simulink model "PubIfDecisionLM_MDL"  (R2020b)
settings: configuration reference "DspaceConfig" (kept outside this file)
PostLoadFcn:
  | if any(exist('dsrtsu_mdlpostloadfcn', 'file') ~= 0), dsrtsu_mdlpostloadfcn('Execute', bdroot); end
InitFcn:
  | , if any(exist('dsmpb_private', 'file') ~= 0), dsmpb_private('dsmpb_mdlclblib', 'Init', bdroot); end,
undefined symbols (not defined in the file or in its folder): OFM_OBJ_FUSIONTYPE_E, OFM_OBJ_MOVINGSTATE_E, OFM_OBJ_ORIENTATION_E, OFM_OBJ_TYPE_E, P_LM_Cyc, P_LM_EMLHistKapRcdBufSize, P_LM_EMLHistTrajBaseDis, P_LM_EMLHistTrajPNum, P_LM_EMLKapCorrMaxThre, P_LM_EMLMinKapThre, P_LM_EMLPathDisDiffThre, P_LM_EMLQuaFiltPar, P_LM_EMLTurnActKapThre, P_LM_EMLValidQuaThre, P_LM_FntPath1Disgap, P_LM_FntPath1MinDis, P_LM_FntPath1Timegap, P_LM_FntPath2Disgap, P_LM_FntPath2MinDis, P_LM_FntPath2Timegap, P_LM_FntPath3Disgap, P_LM_FntPath3MinDis, P_LM_FntPath3Timegap, P_LM_FusBLParFiltP, P_LM_FusEVDifC2Thre, P_LM_FusEVOPath1AllVSLDisThre, P_LM_FusEVOPath1AllVSLLostNumThre, P_LM_FusEVOPath1AllVSLQuaThre, P_LM_FusEVOPath1OTLFacNLC, P_LM_FusOTLQuaThre, P_LM_FusOTLSW, P_LM_FusParC0Index, P_LM_FusParC1Index, P_LM_FusParC2Index, P_LM_FusParC3Index, P_LM_FusVSLQuaThre, P_LM_FusVSLSW, P_LM_FusVSLValidSteerWheerAngThre, P_LM_FusVSLValidVxvThre, P_LM_LaneWidth, P_LM_OTLBufTPInfoEvaFactor, P_LM_OTLObjNum, P_LM_OTLObjSelectAgeThre, P_LM_OTLObjSelectDxAssessVx, P_LM_OTLObjSelectDxThre, P_LM_OTLObjSelectVxThre, P_LM_OTLObjSelectVyAssessDx, P_LM_OTLObjSelectVyThre, P_LM_OTLTrajPntBaseDis, P_LM_OTLTrajStdThre, P_LM_VSLAvailLineNum, P_LM_VSLBLSDiffThre, P_LM_VSLBLSDisRatio, P_LM_VSLFusBLParFiltP_C1, P_LM_VSLFusBLParFiltP_C2, P_LM_VSLFusBLParFiltP_C3, P_LM_VSLFusBLParFiltP_Quality, P_LM_VSLHistTrajBaseDis, P_LM_VSLHistTrajPNum, P_LM_VSLLCC0diff ... (+18)
libraries: simulink x145, LM_LIB x43
(part 14 of 24)

== system PubIfDecisionLM_MDL/Subsystem2/LM_VSL/LM_VSLFntPath/LM_VSL_LineInfoEvalutaion/LM_VSL_BaseLinePCalc3/Subsystem1 ==
  LM_VSLBaseC1 : Inport
  LM_VSLBaseC2 : Inport  Port=2
  LM_VSLBaseC3 : Inport  Port=3
  LM_VSLBaseQuality : Inport  Port=4
  Add{1..3,12} (4 alike) : Sum
  Constant1 : Constant  Value=P_LM_VSLFusBLParFiltP_C2  OutDataTypeStr=single
  Constant10 : Constant  Value=P_LM_VSLFusBLParFiltP_C1  OutDataTypeStr=single
  Constant2 : Constant  Value=P_LM_VSLFusBLParFiltP_C3  OutDataTypeStr=single
  Constant3 : Constant  Value=P_LM_VSLFusBLParFiltP_Quality  OutDataTypeStr=single
  Data Type Conversion : DataTypeConversion  OutDataTypeStr=single
  Product{1..3,17} (4 alike) : Product
  Subtract{1..4} (4 alike) : Sum  Inputs=+-
  Unit Delay{1..4} (4 alike) : UnitDelay  SampleTime=-1  HasFrameUpgradeWarning=on
  LM_VSLBaseC1Filt : Outport
  LM_VSLBaseC2Filt : Outport  Port=2
  LM_VSLBaseC3Filt : Outport  Port=3
  LM_VSLBaseQualityFilt : Outport  Port=4
  wires:
  Data Type Conversion/1 -> LM_VSLBaseQualityFilt/1
  LM_VSLBaseQuality/1 -> Subtract4/1
  Product3/1 -> Add3/1
  Subtract4/1 -> Product3/1
  Unit Delay4/1 -> Subtract4/2, Add3/2
  Constant3/1 -> Product3/2
  Add3/1 -> Unit Delay4/1, Data Type Conversion/1
  Add2/1 -> Unit Delay3/1, LM_VSLBaseC3Filt/1
  Constant2/1 -> Product2/2
  Unit Delay3/1 -> Add2/2, Subtract3/2
  Subtract3/1 -> Product2/1
  Product2/1 -> Add2/1
  LM_VSLBaseC3/1 -> Subtract3/1
  LM_VSLBaseC2/1 -> Subtract1/1
  Product1/1 -> Add1/1
  Subtract1/1 -> Product1/1
  Unit Delay1/1 -> Subtract1/2, Add1/2
  Constant1/1 -> Product1/2
  Constant10/1 -> Product17/2
  Unit Delay2/1 -> Add12/2, Subtract2/2
  Subtract2/1 -> Product17/1
  Product17/1 -> Add12/1
  LM_VSLBaseC1/1 -> Subtract2/1
  Add12/1 -> LM_VSLBaseC1Filt/1, Unit Delay2/1
  Add1/1 -> Unit Delay1/1, LM_VSLBaseC2Filt/1

== system PubIfDecisionLM_MDL/Subsystem2/LM_VSL/LM_VSLFntPath/LM_VSL_LineInfoEvalutaion/LM_VSL_LineInfoEvalutaion/LM_VSL_LineDiffEvalutaion ==
  LM_VSLLineExistVect : Inport
  LM_VSLLineQualityVect : Inport  Port=2
  LM_VSLLineDisFntVect : Inport  Port=3
  LM_ComLineLostNum : Inport  Port=4
  LM_VSLLineC0Vect : Inport  Port=5
  LM_VSLLineC1Vect : Inport  Port=6
  LM_VSLLineC2Vect : Inport  Port=7
  LM_VSLLineC3Vect : Inport  Port=8
  LM_VSLLineMaxQuality : Inport  Port=9
  LM_VSLLineMaxDis : Inport  Port=10
  LM_VSLLineMaxDisIndex : Inport  Port=11
  LM_VSLLineMaxQualityIndex : Inport  Port=12
  Constant : Constant  Value=P_LM_VSLBLSDiffThre  OutDataTypeStr=single
  Constant1 : Constant  Value=P_LM_VSLBLSDisRatio  OutDataTypeStr=single
  LM_VSL_BaseLineSelc : MATLAB Function  TreatAsAtomicUnit=on
  LM_VSL_DiffMaxLineEvaluation3 : MATLAB Function  TreatAsAtomicUnit=on
  Terminator : Terminator
  "Diffnum " : Outport
  LM_VSLDiffValid : Outport  Port=2
  LM_VSLBLFntDis : Outport  Port=3
  wires:
  Constant1/1 -> LM_VSL_DiffMaxLineEvaluation3/11(P_LM_VSLBLSDisRatio)
  Constant/1 -> LM_VSL_DiffMaxLineEvaluation3/10(P_LM_VSLBLSDiffThre)
  LM_VSL_DiffMaxLineEvaluation3/2(LM_VSLDiffValue) -> Terminator/1  "LM_VSLDiffValue"
  LM_VSL_BaseLineSelc/2(LM_VSLBLFntDis) -> LM_VSL_DiffMaxLineEvaluation3/2(LM_VSLBLFntDis), LM_VSLBLFntDis/1
  LM_VSL_DiffMaxLineEvaluation3/3(Diffnum) -> "Diffnum "/1
  [LM_VSLLineDisFntVect] -> LM_VSL_DiffMaxLineEvaluation3/9(LM_VSLLineDisFntVect)
  LM_VSL_DiffMaxLineEvaluation3/1(LM_VSLDiffValid) -> LM_VSLDiffValid/1
  LM_VSLLineC2Vect/1 -> LM_VSL_DiffMaxLineEvaluation3/7(LM_VSLLineC2Vect)
  LM_VSLLineQualityVect/1 -> LM_VSL_BaseLineSelc/1(LM_VSLLineQualityVect)
  LM_ComLineLostNum/1 -> LM_VSL_DiffMaxLineEvaluation3/5(LM_ComLineLostNum)
  LM_VSLLineExistVect/1 -> LM_VSL_BaseLineSelc/7(LM_VSLLineExistVect), LM_VSL_DiffMaxLineEvaluation3/3(LM_VSLLineExistVect)
  LM_VSL_BaseLineSelc/1(LM_VSLBLIndex) -> LM_VSL_DiffMaxLineEvaluation3/1(LM_VSLBLIndex)  "LM_VSLBLIndex"
  LM_VSLLineC0Vect/1 -> LM_VSL_DiffMaxLineEvaluation3/4(LM_VSLLineC0Vect)
  LM_VSLLineC1Vect/1 -> LM_VSL_DiffMaxLineEvaluation3/6(LM_VSLLineC1Vect)
  LM_VSLLineC3Vect/1 -> LM_VSL_DiffMaxLineEvaluation3/8(LM_VSLLineC3Vect)
  LM_VSLLineDisFntVect/1 -> LM_VSL_BaseLineSelc/2(LM_VSLLineDisFntVect), [LM_VSLLineDisFntVect]
  LM_VSLLineMaxDis/1 -> LM_VSL_BaseLineSelc/3(LM_VSLLineMaxDis)
  LM_VSLLineMaxDisIndex/1 -> LM_VSL_BaseLineSelc/4(LM_VSLLineMaxDisIndex)
  LM_VSLLineMaxQuality/1 -> LM_VSL_BaseLineSelc/5(LM_VSLLineMaxQuality)
  LM_VSLLineMaxQualityIndex/1 -> LM_VSL_BaseLineSelc/6(LM_VSLLineMaxQualityIndex)

== system PubIfDecisionLM_MDL/Subsystem2/LM_VSL/LM_VSLFntPath/LM_VSL_LineInfoEvalutaion/LM_VSL_LineInfoEvalutaion/LM_VSL_LineDisEvaluation ==
  LM_ComAllLineLost_flg : Inport
  LM_VSLLineExistVect : Inport  Port=2
  LM_VSLLineDisFntVect : Inport  Port=3
  If : If  IfExpression=u1 == 1
  If Action Subsystem : Subsystem  TreatAsAtomicUnit=on
  If Action Subsystem1 : Subsystem  TreatAsAtomicUnit=on
  Merge{,1..3} (4 alike) : Merge
  Terminator1 : Terminator
  Terminator2 : Terminator
  LM_VSLLineMaxDis : Outport
  LM_VSLLineMaxDisIndex : Outport  Port=2
  wires:
  Merge3/1 -> Terminator2/1
  If Action Subsystem1/4(LM_VSLLineMeanDis) -> Merge3/2
  If Action Subsystem/4(LM_VSLLineMeanDis) -> Merge3/1
  LM_ComAllLineLost_flg/1 -> If/1
  If/1 -> If Action Subsystem/Action
  If/2 -> If Action Subsystem1/Action
  LM_VSLLineExistVect/1 -> If Action Subsystem1/1(LM_VSLLineExistVect)
  LM_VSLLineDisFntVect/1 -> If Action Subsystem1/2(LM_VSLLineDisFntVect)
  If Action Subsystem/1(LM_VSLLineMaxDis) -> Merge/1
  If Action Subsystem1/1(LM_VSLLineMaxDis) -> Merge/2
  Merge/1 -> LM_VSLLineMaxDis/1
  If Action Subsystem1/2(LM_VSLLineMaxDisIndex) -> Merge1/2
  If Action Subsystem/2(LM_VSLLineMaxDisIndex) -> Merge1/1
  Merge1/1 -> LM_VSLLineMaxDisIndex/1
  If Action Subsystem/3(LM_VSLLineDisSortIndexVect) -> Merge2/1
  Merge2/1 -> Terminator1/1
  If Action Subsystem1/3(LM_VSLLineDisSortIndexVect) -> Merge2/2

== system PubIfDecisionLM_MDL/Subsystem2/LM_VSL/LM_VSLFntPath/LM_VSL_LineInfoEvalutaion/LM_VSL_LineInfoEvalutaion/LM_VSL_LineQualityEvalutaion ==
  LM_ComAllLineLost_flg : Inport
  LM_VSLLineExistVect : Inport  Port=2
  LM_VSLLineQualityVect : Inport  Port=3
  If : If  IfExpression=u1 == 1
  If Action Subsystem : Subsystem  TreatAsAtomicUnit=on
  If Action Subsystem1 : Subsystem  TreatAsAtomicUnit=on
  LM_VSLMinQualityLineValidJudge : Subsystem
  Merge{,1..5} (6 alike) : Merge
  Terminator2 : Terminator
  LM_VSLLineMinQualityIndex : Outport
  LM_VSLLineMaxQualityIndex : Outport  Port=2
  LM_VSLLineMaxQuality : Outport  Port=3
  LM_VSLMinQualityLineValid : Outport  Port=4
  wires:
  If/1 -> If Action Subsystem/Action
  If/2 -> If Action Subsystem1/Action
  LM_ComAllLineLost_flg/1 -> If/1
  LM_VSLLineQualityVect/1 -> If Action Subsystem1/2(LM_VSLLineQualityVect)
  LM_VSLLineExistVect/1 -> If Action Subsystem1/1(LM_VSLLineExistVect)
  If Action Subsystem/1(LM_VSLLineMaxQuality) -> Merge/1
  If Action Subsystem/2(LM_VSLLineMaxQualityIndex) -> Merge1/1
  If Action Subsystem/4(LM_VSLLineMinQuality) -> Merge2/1
  If Action Subsystem/3(LM_VSLLineMinQualityIndex) -> Merge3/1
  If Action Subsystem/5(LM_VSLLineMeanQuality) -> Merge4/1
  If Action Subsystem/6(LM_VSLLineQualityVar) -> Merge5/1
  Merge/1 -> LM_VSLLineMaxQuality/1  "LM_VSLLineMaxQuality"
  Merge1/1 -> LM_VSLLineMaxQualityIndex/1  "LM_VSLLineMaxQualityIndex"
  Merge2/1 -> LM_VSLMinQualityLineValidJudge/1(LM_VSLLineMinQuality)  "LM_VSLLineMinQuality"
  Merge3/1 -> LM_VSLLineMinQualityIndex/1  "LM_VSLLineMinQualityIndex"
  Merge4/1 -> LM_VSLMinQualityLineValidJudge/2(LM_VSLLineMeanQuality)  "LM_VSLLineMeanQuality"
  Merge5/1 -> Terminator2/1
  If Action Subsystem1/1(LM_VSLLineMaxQuality) -> Merge/2
  If Action Subsystem1/2(LM_VSLLineMaxQualityIndex) -> Merge1/2
  If Action Subsystem1/4(LM_VSLLineMinQuality) -> Merge2/2
  If Action Subsystem1/3(LM_VSLLineMinQualityIndex) -> Merge3/2
  If Action Subsystem1/5(LM_VSLLineMeanQuality) -> Merge4/2
  If Action Subsystem1/6(LM_VSLLineQualityVar) -> Merge5/2
  LM_VSLMinQualityLineValidJudge/1(LM_VSLMinQualityLineValid) -> LM_VSLMinQualityLineValid/1

== system PubIfDecisionLM_MDL/Subsystem2/LM_VSL/LM_VSLRearPath/LM_VSLHistLineInfoCoordinateConvert/If Action Subsystem/For Each Subsystem ==
  LM_EMLOffsetX : Inport
  LM_EMLOffsetY : Inport  Port=2
  LM_EMLOffsetAng : Inport  Port=3
  LM_VSLLRC0HistInfoXK1 : Inport  Port=4  Partition=on  PartitionDimension=1  PartitionWidth=1  PartitionOffset=0
  LM_VSLLRC0HistInfoYK1 : Inport  Port=5  Partition=on  PartitionDimension=1  PartitionWidth=1  PartitionOffset=0
  LM_VSLRLC0HistInfoXK1 : Inport  Port=6  Partition=on  PartitionDimension=1  PartitionWidth=1  PartitionOffset=0
  LM_VSLRLC0HistInfoYK1 : Inport  Port=7  Partition=on  PartitionDimension=1  PartitionWidth=1  PartitionOffset=0
  For Each : ForEach  DisableCoverage=on
  LM_VSL_LRC0HistInfoConvert : Subsystem
  LM_VSL_RLC0HistInfoConvert : Subsystem
  LM_VSLLRC0HistInfoXK1Adju : Outport  ConcatenationDimension=1
  LM_VSLLRC0HistInfoYK1Adju : Outport  Port=2  ConcatenationDimension=1
  LM_VSLRLC0HistInfoXK1Adju : Outport  Port=3  ConcatenationDimension=1
  LM_VSLRLC0HistInfoYK1Adju : Outport  Port=4  ConcatenationDimension=1
  wires:
  LM_EMLOffsetX/1 -> LM_VSL_RLC0HistInfoConvert/3(LM_EgoVehOffsetX), LM_VSL_LRC0HistInfoConvert/3(LM_EgoVehOffsetX)
  LM_EMLOffsetY/1 -> LM_VSL_RLC0HistInfoConvert/4(LM_EgoVehOffsetY), LM_VSL_LRC0HistInfoConvert/4(LM_EgoVehOffsetY)
  LM_EMLOffsetAng/1 -> LM_VSL_RLC0HistInfoConvert/5(LM_EgoVehOffsetAng), LM_VSL_LRC0HistInfoConvert/5(LM_EgoVehOffsetAng)
  LM_VSL_LRC0HistInfoConvert/1(LM_VSLLLC0HistInfoXK1Adju) -> LM_VSLLRC0HistInfoXK1Adju/1
  LM_VSL_LRC0HistInfoConvert/2(LM_VSLLLC0HistInfoYK1Adju) -> LM_VSLLRC0HistInfoYK1Adju/1
  LM_VSL_RLC0HistInfoConvert/2(LM_VSLLLC0HistInfoYK1Adju) -> LM_VSLRLC0HistInfoYK1Adju/1
  LM_VSL_RLC0HistInfoConvert/1(LM_VSLLLC0HistInfoXK1Adju) -> LM_VSLRLC0HistInfoXK1Adju/1
  LM_VSLLRC0HistInfoYK1/1 -> LM_VSL_LRC0HistInfoConvert/2(LM_VSLLRC0HistInfoYK1)
  LM_VSLLRC0HistInfoXK1/1 -> LM_VSL_LRC0HistInfoConvert/1(LM_VSLLRC0HistInfoXK1)
  LM_VSLRLC0HistInfoYK1/1 -> LM_VSL_RLC0HistInfoConvert/2(LM_VSLRLC0HistInfoYK1)
  LM_VSLRLC0HistInfoXK1/1 -> LM_VSL_RLC0HistInfoConvert/1(LM_VSLRLC0HistInfoXK1)

== system PubIfDecisionLM_MDL/Subsystem2/DIR/DrivingIntentionRecognition1/DIR_LaneChangeProbCalc/DIR_LaneChangeLeftProbCalc/If Action Subsystem/DIR_LaneChgLeProbByC1 ==
  LM_VSLFntPathBaseC1 : Inport
  Constant5 : Constant  Value=-0.035  OutDataTypeStr=single
  Relational Operator5 : RelationalOperator  Operator=<=  OutDataTypeStr=boolean  RndMeth=Nearest
  DIR_LaneChgLeByLineC1Valid : Outport
  wires:
  Constant5/1 -> Relational Operator5/2
  LM_VSLFntPathBaseC1/1 -> Relational Operator5/1
  Relational Operator5/1 -> DIR_LaneChgLeByLineC1Valid/1  "DIR_LaneChgLeByLineC1Valid"

== system PubIfDecisionLM_MDL/Subsystem2/DIR/DrivingIntentionRecognition1/DIR_LaneChangeProbCalc/DIR_LaneChangeLeftProbCalc/If Action Subsystem/DIR_LaneChgLeProbByLaneInfo ==
  LM_LRC0 : Inport
  LM_RLC0 : Inport  Port=2
  DIR_LaneC0DifCalc : Subsystem
  DIR_LaneChgLeProbCalcByLaneBorder : Subsystem
  Unit Delay : UnitDelay  SampleTime=-1  HasFrameUpgradeWarning=on
  DIR_LC2LeProbByLaneBorder : Outport
  wires:
  DIR_LaneC0DifCalc/1(DIR_LaneC0Dif) -> Unit Delay/1, DIR_LaneChgLeProbCalcByLaneBorder/1(DIR_LaneC0Dif)
  Unit Delay/1 -> DIR_LaneC0DifCalc/1(DIR_LaneC0DifK1)
  LM_LRC0/1 -> DIR_LaneChgLeProbCalcByLaneBorder/2(LM_LRC0), DIR_LaneC0DifCalc/2(LM_LRC0)
  LM_RLC0/1 -> DIR_LaneC0DifCalc/3(LM_RLC0)
  DIR_LaneChgLeProbCalcByLaneBorder/1(DIR_LC2LeProbByLaneBorder) -> DIR_LC2LeProbByLaneBorder/1

== system PubIfDecisionLM_MDL/Subsystem2/DIR/DrivingIntentionRecognition1/DIR_LaneChangeProbCalc/DIR_LaneChangeLeftProbCalc/If Action Subsystem/DIR_LaneChgLeProbByLeftTurnSWSts ==
  LeftTurnSWSts : Inport
  Constant : Constant  OutDataTypeStr=uint8
  Constant1 : Constant  OutDataTypeStr=single
  Constant2 : Constant  Value=0  OutDataTypeStr=single
  Relational Operator : RelationalOperator  Operator===  OutDataTypeStr=boolean  RndMeth=Simplest
  Switch : Switch  Criteria=u2 ~= 0
  DIR_LC2LeProbByTurnLampSts : Outport
  wires:
  Switch/1 -> DIR_LC2LeProbByTurnLampSts/1  "DIR_LC2LeProbByTurnLampSts"
  Constant2/1 -> Switch/3
  Constant/1 -> Relational Operator/2
  Relational Operator/1 -> Switch/2
  LeftTurnSWSts/1 -> Relational Operator/1
  Constant1/1 -> Switch/1

== system PubIfDecisionLM_MDL/Subsystem2/DIR/DrivingIntentionRecognition1/DIR_LaneChangeProbCalc/DIR_LaneChangeLeftProbCalc/If Action Subsystem/DIR_LaneChgLeProbCalc ==
  DIR_LC2LeProbBySteer : Inport
  DIR_LC2LeProbByLaneBorder : Inport  Port=2
  DIR_LC2LeProbByTurnLampSts : Inport  Port=3
  DIR_LaneChgLeByLineC1Valid : Inport  Port=4
  Add : Sum
  Add1 : Sum
  Constant : Constant  Value=2  OutDataTypeStr=single
  Constant1 : Constant  Value=0.1  OutDataTypeStr=single
  Constant2 : Constant  Value=0.25  OutDataTypeStr=single
  Constant3 : Constant  Value=0.75  OutDataTypeStr=single
  Constant4 : Constant  Value=0.75  OutDataTypeStr=single
  Divide : Product  Inputs=*/
  Logical Operator : Logic  AllPortsSameDT=off  OutDataTypeStr=boolean
  MinMax : MinMax  Inputs=2
  Product : Product
  Relational Operator : RelationalOperator  Operator=>  OutDataTypeStr=boolean  RndMeth=Simplest
  Relational Operator1 : RelationalOperator  OutDataTypeStr=boolean  RndMeth=Simplest
  Switch : Switch  Criteria=u2 ~= 0
  DIR_tLC2LeValid : Outport
  wires:
  DIR_LC2LeProbBySteer/1 -> Add/1
  DIR_LC2LeProbByLaneBorder/1 -> Add/2
  Add/1 -> Divide/1
  Constant/1 -> Divide/2
  Divide/1 -> MinMax/1
  DIR_LC2LeProbByTurnLampSts/1 -> MinMax/2
  Constant1/1 -> Relational Operator/2
  Relational Operator/1 -> Switch/2
  MinMax/1 -> Switch/3, Product/1, Relational Operator/1
  Constant2/1 -> Product/2
  Product/1 -> Add1/1
  Constant3/1 -> Add1/2
  Add1/1 -> Switch/1
  Switch/1 -> Relational Operator1/1  "DIR_LC2LeProb"
  Constant4/1 -> Relational Operator1/2
  Logical Operator/1 -> DIR_tLC2LeValid/1  "DIR_tLC2LeValid"
  DIR_LaneChgLeByLineC1Valid/1 -> Logical Operator/1
  Relational Operator1/1 -> Logical Operator/2  "DIR_tLC2LeValid"

== system PubIfDecisionLM_MDL/Subsystem2/DIR/DrivingIntentionRecognition1/DIR_LaneChangeProbCalc/DIR_LaneChangeLeftProbCalc/If Action Subsystem/DIR_LaneChgLeProbCalcBySteer ==
  DIR_LeftTurnLampOnTime : Inport
  SteerWheelAngle : Inport  Port=2
  SteerWheelAngleSign : Inport  Port=3
  DIR_LaneChg2LeftProbCalcBySteer : Subsystem
  DIR_LaneChg2LeftProbCalcBySteerWheelAng : Subsystem
  DIR_LaneChg2LeftProbCalcByTurnLampOnTime : Subsystem
  DIR_LC2LeProbBySteer : Outport
  wires:
  DIR_LaneChg2LeftProbCalcBySteerWheelAng/1(DIR_LC2LeProbBySteerWheelAng) -> DIR_LaneChg2LeftProbCalcBySteer/1(DIR_LC2LeProbBySteerWheelAng)
  DIR_LaneChg2LeftProbCalcByTurnLampOnTime/1(DIR_LC2LeProbBytTurnLamp) -> DIR_LaneChg2LeftProbCalcBySteer/2(DIR_LC2LeProbBytTurnLamp)
  DIR_LeftTurnLampOnTime/1 -> DIR_LaneChg2LeftProbCalcByTurnLampOnTime/1(DIR_LeftTurnLampOnTime)
  DIR_LaneChg2LeftProbCalcBySteer/1(DIR_LC2LeProbBySteer) -> DIR_LC2LeProbBySteer/1
  SteerWheelAngle/1 -> DIR_LaneChg2LeftProbCalcBySteerWheelAng/1(SteerWheelAngle)
  SteerWheelAngleSign/1 -> DIR_LaneChg2LeftProbCalcBySteerWheelAng/2(SteerWheelAngleSign)

== system PubIfDecisionLM_MDL/Subsystem2/DIR/DrivingIntentionRecognition1/DIR_LaneChangeProbCalc/DIR_LaneChangeLeftProbCalc/If Action Subsystem1/DIR_LaneChgLeProbByLaneInfo ==
  LM_LRC0 : Inport
  LM_RLC0 : Inport  Port=2
  Abs : Abs
  Abs1 : Abs
  Abs2 : Abs
  Add : Sum
  Constant : Constant  Value=0.8  OutDataTypeStr=single
  Constant1 : Constant  Value=0.05  OutDataTypeStr=single
  Constant2 : Constant  Value=0.1  OutDataTypeStr=single
  Constant3 : Constant  Value=0.6  OutDataTypeStr=single
  Constant4 : Constant  Value=0  OutDataTypeStr=single
  Logical Operator : Logic  Operator=OR  AllPortsSameDT=off  OutDataTypeStr=boolean
  Logical Operator1 : Logic  AllPortsSameDT=off  OutDataTypeStr=boolean
  Logical Operator2 : Logic  Operator=OR  AllPortsSameDT=off  OutDataTypeStr=boolean
  Logical Operator3 : Logic  AllPortsSameDT=off  OutDataTypeStr=boolean
  MinMax : MinMax  Function=max
  Product : Product
  Relational Operator{,1..3} (4 alike) : RelationalOperator  Operator=>  OutDataTypeStr=boolean  RndMeth=Simplest
  Relational Operator4 : RelationalOperator  Operator=<  OutDataTypeStr=boolean  RndMeth=Simplest
  Subtract : Sum  Inputs=+-
  Subtract1 : Sum  Inputs=+-
  Tapped Delay : simulink/Discrete/Tapped Delay  vinit=0.0  samptime=-1  NumDelays=5  DelayOrder=Oldest  includeCurrent=off
  Unit Delay : UnitDelay  SampleTime=-1  HasFrameUpgradeWarning=on
  Unit Delay1 : UnitDelay  SampleTime=-1  HasFrameUpgradeWarning=on
  DIR_LaneChgLeByLaneBorderValid : Outport
  wires:
  Logical Operator3/1 -> DIR_LaneChgLeByLaneBorderValid/1  "DIR_LaneChgLeByLaneBorderValid"
  LM_LRC0/1 -> Add/1, Product/1
  LM_RLC0/1 -> Product/2, Add/2
  Add/1 -> Abs/1
  Unit Delay1/1 -> Subtract1/2
  Unit Delay/1 -> Unit Delay1/1, Subtract/2
  Constant/1 -> Relational Operator/2
  Abs/1 -> Subtract1/1, Subtract/1, Relational Operator/1, Unit Delay/1
  Subtract/1 -> Abs1/1
  Abs1/1 -> Tapped Delay/1, Relational Operator1/1
  Subtract1/1 -> Abs2/1
  Abs2/1 -> Relational Operator2/1
  Constant1/1 -> Relational Operator1/2
  Constant2/1 -> Relational Operator2/2
  Relational Operator1/1 -> Logical Operator/1
  Relational Operator2/1 -> Logical Operator/2
  Tapped Delay/1 -> MinMax/1
  MinMax/1 -> Relational Operator3/1
  Constant3/1 -> Relational Operator3/2
  Product/1 -> Relational Operator4/1
  Constant4/1 -> Relational Operator4/2
  Relational Operator4/1 -> Logical Operator1/1
  Relational Operator/1 -> Logical Operator1/2
  Relational Operator3/1 -> Logical Operator2/1
  Logical Operator/1 -> Logical Operator2/2
  Logical Operator1/1 -> Logical Operator3/1
  Logical Operator2/1 -> Logical Operator3/2

== system PubIfDecisionLM_MDL/Subsystem2/DIR/DrivingIntentionRecognition1/DIR_LaneChangeProbCalc/DIR_LaneChangeLeftProbCalc/If Action Subsystem1/DIR_LaneChgLeProbByLaneInfo1 ==
  LM_VSLFntPathBaseC1 : Inport
  Constant5 : Constant  Value=-0.035  OutDataTypeStr=single
  Relational Operator5 : RelationalOperator  Operator=<=  OutDataTypeStr=boolean  RndMeth=Nearest
  DIR_LaneChgLeByLineC1Valid : Outport
  wires:
  Constant5/1 -> Relational Operator5/2
  LM_VSLFntPathBaseC1/1 -> Relational Operator5/1
  Relational Operator5/1 -> DIR_LaneChgLeByLineC1Valid/1  "DIR_LaneChgLeByLineC1Valid"

== system PubIfDecisionLM_MDL/Subsystem2/DIR/DrivingIntentionRecognition1/DIR_LaneChangeProbCalc/DIR_LaneChangeLeftProbCalc/If Action Subsystem1/DIR_LaneChgLeProbCalc ==
  DIR_LC2LeProbBySteer : Inport
  DIR_LC2LeProbByLaneBorder : Inport  Port=2
  DIR_LaneChgLeByLineC1Valid : Inport  Port=3
  Logical Operator : Logic  Operator=OR  AllPortsSameDT=off  OutDataTypeStr=boolean
  Logical Operator1 : Logic  AllPortsSameDT=off  OutDataTypeStr=boolean
  DIR_tLC2LeValid : Outport
  wires:
  Logical Operator1/1 -> DIR_tLC2LeValid/1  "DIR_tLC2LeValid"
  DIR_LC2LeProbBySteer/1 -> Logical Operator/1
  DIR_LC2LeProbByLaneBorder/1 -> Logical Operator/2
  Logical Operator/1 -> Logical Operator1/1
  DIR_LaneChgLeByLineC1Valid/1 -> Logical Operator1/2

== system PubIfDecisionLM_MDL/Subsystem2/DIR/DrivingIntentionRecognition1/DIR_LaneChangeProbCalc/DIR_LaneChangeLeftProbCalc/If Action Subsystem1/DIR_LaneChgLeProbCalcBySteer ==
  SteerWheelAngle : Inport
  SteerWheelAngleSign : Inport  Port=2
  DIR_EgoVehOnLineValid : Inport  Port=3
  vxvRefMs : Inport  Port=4
  If : If  IfExpression=u1 ~= 0
  If Action Subsystem : Subsystem  TreatAsAtomicUnit=on
  If Action Subsystem1 : Subsystem  TreatAsAtomicUnit=on
  Merge : Merge
  DIR_LaneChgLeBySteerValid : Outport
  wires:
  DIR_EgoVehOnLineValid/1 -> If/1
  If/1 -> If Action Subsystem/Action
  If/2 -> If Action Subsystem1/Action
  SteerWheelAngle/1 -> If Action Subsystem1/1(SteerWheelAngle), If Action Subsystem/1(SteerWheelAngle)
  SteerWheelAngleSign/1 -> If Action Subsystem1/2(SteerWheelAngleSign), If Action Subsystem/2(SteerWheelAngleSign)
  vxvRefMs/1 -> If Action Subsystem1/3(vxvRefMs), If Action Subsystem/3(vxvRefMs)
  If Action Subsystem/1(DIR_LaneChgLeBySteerValid) -> Merge/1
  If Action Subsystem1/1(DIR_LaneChgLeBySteerValid) -> Merge/2
  Merge/1 -> DIR_LaneChgLeBySteerValid/1  "DIR_LaneChgLeBySteerValid"

== system PubIfDecisionLM_MDL/Subsystem2/DIR/DrivingIntentionRecognition1/DIR_LaneChangeProbCalc/DIR_LaneChangeRightProbCalc/If Action Subsystem/DIR_LaneChgLeProbByLaneInfo ==
  LM_LRC0 : Inport
  LM_RLC0 : Inport  Port=2
  DIR_LaneC0DifCalc : Subsystem
  DIR_LaneChgLeProbCalcByLaneBorder : Subsystem
  Unit Delay : UnitDelay  SampleTime=-1  HasFrameUpgradeWarning=on
  DIR_LC2LeProbByLaneBorder : Outport
  wires:
  DIR_LaneChgLeProbCalcByLaneBorder/1(DIR_LC2RigProbByLaneBorder) -> DIR_LC2LeProbByLaneBorder/1
  LM_RLC0/1 -> DIR_LaneC0DifCalc/3(LM_RLC0)
  LM_LRC0/1 -> DIR_LaneC0DifCalc/2(LM_LRC0), DIR_LaneChgLeProbCalcByLaneBorder/2(LM_LRC0)
  Unit Delay/1 -> DIR_LaneC0DifCalc/1(DIR_LaneC0DifK1)
  DIR_LaneC0DifCalc/1(DIR_LaneC0Dif) -> DIR_LaneChgLeProbCalcByLaneBorder/1(DIR_LaneC0Dif), Unit Delay/1

== system PubIfDecisionLM_MDL/Subsystem2/DIR/DrivingIntentionRecognition1/DIR_LaneChangeProbCalc/DIR_LaneChangeRightProbCalc/If Action Subsystem/DIR_LaneChgLeProbByLaneInfo1 ==
  LM_VSLFntPathBaseC1 : Inport
  Constant5 : Constant  Value=0.015  OutDataTypeStr=single
  Relational Operator5 : RelationalOperator  Operator=>  OutDataTypeStr=boolean  RndMeth=Nearest
  DIR_LaneChgRigByLineC1Valid : Outport
  wires:
  Relational Operator5/1 -> DIR_LaneChgRigByLineC1Valid/1  "DIR_LaneChgRigByLineC1Valid"
  LM_VSLFntPathBaseC1/1 -> Relational Operator5/1
  Constant5/1 -> Relational Operator5/2

== system PubIfDecisionLM_MDL/Subsystem2/DIR/DrivingIntentionRecognition1/DIR_LaneChangeProbCalc/DIR_LaneChangeRightProbCalc/If Action Subsystem/DIR_LaneChgLeProbByLeftTurnSWSts ==
  RightTurnSWSts : Inport
  Constant : Constant  OutDataTypeStr=uint8
  Constant1 : Constant  OutDataTypeStr=single
  Constant2 : Constant  Value=0  OutDataTypeStr=single
  Relational Operator : RelationalOperator  Operator===  OutDataTypeStr=boolean  RndMeth=Simplest
  Switch : Switch  Criteria=u2 ~= 0
  DIR_LC2RigProbByTurnLampSts : Outport
  wires:
  Constant1/1 -> Switch/1
  RightTurnSWSts/1 -> Relational Operator/1
  Relational Operator/1 -> Switch/2
  Constant/1 -> Relational Operator/2
  Constant2/1 -> Switch/3
  Switch/1 -> DIR_LC2RigProbByTurnLampSts/1  "DIR_LC2RigProbByTurnLampSts"

== system PubIfDecisionLM_MDL/Subsystem2/DIR/DrivingIntentionRecognition1/DIR_LaneChangeProbCalc/DIR_LaneChangeRightProbCalc/If Action Subsystem/DIR_LaneChgLeProbCalc ==
  DIR_LC2RigProbBySteer : Inport
  DIR_LC2RigProbByLaneBorder : Inport  Port=2
  DIR_LC2RigProbByTurnLampSts : Inport  Port=3
  DIR_LaneChgRigByLineC1Valid : Inport  Port=4
  Add : Sum
  Add1 : Sum
  Constant : Constant  Value=2  OutDataTypeStr=single
  Constant1 : Constant  Value=0.1  OutDataTypeStr=single
  Constant2 : Constant  Value=0.25  OutDataTypeStr=single
  Constant3 : Constant  Value=0.75  OutDataTypeStr=single
  Constant4 : Constant  Value=0.75  OutDataTypeStr=single
  Divide : Product  Inputs=*/
  Logical Operator : Logic  AllPortsSameDT=off  OutDataTypeStr=boolean
  MinMax : MinMax  Inputs=2
  Product : Product
  Relational Operator : RelationalOperator  Operator=>  OutDataTypeStr=boolean  RndMeth=Simplest
  Relational Operator1 : RelationalOperator  OutDataTypeStr=boolean  RndMeth=Simplest
  Switch : Switch  Criteria=u2 ~= 0
  DIR_tLC2RigValid : Outport
  wires:
  Relational Operator1/1 -> Logical Operator/2  "DIR_tLC2RigValid"
  Constant4/1 -> Relational Operator1/2
  Switch/1 -> Relational Operator1/1  "DIR_LC2LeProb"
  Add1/1 -> Switch/1
  Constant3/1 -> Add1/2
  Product/1 -> Add1/1
  Constant2/1 -> Product/2
  MinMax/1 -> Relational Operator/1, Product/1, Switch/3
  Relational Operator/1 -> Switch/2
  Constant1/1 -> Relational Operator/2
  DIR_LC2RigProbByTurnLampSts/1 -> MinMax/2
  Divide/1 -> MinMax/1
  Constant/1 -> Divide/2
  Add/1 -> Divide/1
  DIR_LC2RigProbByLaneBorder/1 -> Add/2
  DIR_LC2RigProbBySteer/1 -> Add/1
  DIR_LaneChgRigByLineC1Valid/1 -> Logical Operator/1
  Logical Operator/1 -> DIR_tLC2RigValid/1  "DIR_tLC2RigValid"

== system PubIfDecisionLM_MDL/Subsystem2/DIR/DrivingIntentionRecognition1/DIR_LaneChangeProbCalc/DIR_LaneChangeRightProbCalc/If Action Subsystem/DIR_LaneChgLeProbCalcBySteer ==
  DIR_RightTurnLampOnTime : Inport
  SteerWheelAngle : Inport  Port=2
  SteerWheelAngleSign : Inport  Port=3
  DIR_LaneChg2LeftProbCalcBySteer : Subsystem
  DIR_LaneChg2LeftProbCalcBySteerWheelAng : Subsystem
  DIR_LaneChg2LeftProbCalcByTurnLampOnTime : Subsystem
  DIR_LC2LeProbBySteer : Outport
  wires:
  SteerWheelAngleSign/1 -> DIR_LaneChg2LeftProbCalcBySteerWheelAng/2(SteerWheelAngleSign)
  SteerWheelAngle/1 -> DIR_LaneChg2LeftProbCalcBySteerWheelAng/1(SteerWheelAngle)
  DIR_LaneChg2LeftProbCalcBySteer/1(DIR_LC2RigProbBySteer) -> DIR_LC2LeProbBySteer/1
  DIR_RightTurnLampOnTime/1 -> DIR_LaneChg2LeftProbCalcByTurnLampOnTime/1(DIR_RightTurnLampOnTime)
  DIR_LaneChg2LeftProbCalcByTurnLampOnTime/1(DIR_LC2RigProbBytTurnLamp) -> DIR_LaneChg2LeftProbCalcBySteer/2(DIR_LC2RigProbBytTurnLamp)
  DIR_LaneChg2LeftProbCalcBySteerWheelAng/1(DIR_LC2RigProbBySteerWheelAng) -> DIR_LaneChg2LeftProbCalcBySteer/1(DIR_LC2RigProbBySteerWheelAng)

== system PubIfDecisionLM_MDL/Subsystem2/DIR/DrivingIntentionRecognition1/DIR_LaneChangeProbCalc/DIR_LaneChangeRightProbCalc/If Action Subsystem1/DIR_LaneChgLeProbByLaneInfo ==
  LM_LRC0 : Inport
  LM_RLC0 : Inport  Port=2
  Abs : Abs
  Abs1 : Abs
  Abs2 : Abs
  Add : Sum
  Constant : Constant  Value=0.6  OutDataTypeStr=single
  Constant1 : Constant  Value=0.05  OutDataTypeStr=single
  Constant2 : Constant  Value=0.1  OutDataTypeStr=single
  Constant3 : Constant  Value=0.6  OutDataTypeStr=single
  Constant4 : Constant  Value=0  OutDataTypeStr=single
  Logical Operator : Logic  Operator=OR  AllPortsSameDT=off  OutDataTypeStr=boolean
  Logical Operator1 : Logic  AllPortsSameDT=off  OutDataTypeStr=boolean
  Logical Operator2 : Logic  Operator=OR  AllPortsSameDT=off  OutDataTypeStr=boolean
  Logical Operator3 : Logic  AllPortsSameDT=off  OutDataTypeStr=boolean
  MinMax : MinMax  Function=max
  Product : Product
  Relational Operator{,1..3} (4 alike) : RelationalOperator  Operator=>  OutDataTypeStr=boolean  RndMeth=Simplest
  Relational Operator4 : RelationalOperator  Operator=<  OutDataTypeStr=boolean  RndMeth=Simplest
  Subtract : Sum  Inputs=+-
  Subtract1 : Sum  Inputs=+-
  Tapped Delay : simulink/Discrete/Tapped Delay  vinit=0.0  samptime=-1  NumDelays=5  DelayOrder=Oldest  includeCurrent=off
  Unit Delay : UnitDelay  SampleTime=-1  HasFrameUpgradeWarning=on
  Unit Delay1 : UnitDelay  SampleTime=-1  HasFrameUpgradeWarning=on
  DIR_LaneChgRigByLaneBorderValid : Outport
  wires:
  Logical Operator2/1 -> Logical Operator3/2
  Logical Operator1/1 -> Logical Operator3/1
  Logical Operator/1 -> Logical Operator2/2
  Relational Operator3/1 -> Logical Operator2/1
  Relational Operator/1 -> Logical Operator1/2
  Relational Operator4/1 -> Logical Operator1/1
  Constant4/1 -> Relational Operator4/2
  Product/1 -> Relational Operator4/1
  Constant3/1 -> Relational Operator3/2
  MinMax/1 -> Relational Operator3/1
  Tapped Delay/1 -> MinMax/1
  Relational Operator2/1 -> Logical Operator/2
  Relational Operator1/1 -> Logical Operator/1
  Constant2/1 -> Relational Operator2/2
  Constant1/1 -> Relational Operator1/2
  Abs2/1 -> Relational Operator2/1
  Subtract1/1 -> Abs2/1
  Abs1/1 -> Relational Operator1/1, Tapped Delay/1
  Subtract/1 -> Abs1/1
  Abs/1 -> Unit Delay/1, Relational Operator/1, Subtract/1, Subtract1/1
  Constant/1 -> Relational Operator/2
  Unit Delay/1 -> Subtract/2, Unit Delay1/1
  Unit Delay1/1 -> Subtract1/2
  Add/1 -> Abs/1
  LM_RLC0/1 -> Add/2, Product/2
  LM_LRC0/1 -> Product/1, Add/1
  Logical Operator3/1 -> DIR_LaneChgRigByLaneBorderValid/1  "DIR_LaneChgRigByLaneBorderValid"

== system PubIfDecisionLM_MDL/Subsystem2/DIR/DrivingIntentionRecognition1/DIR_LaneChangeProbCalc/DIR_LaneChangeRightProbCalc/If Action Subsystem1/DIR_LaneChgLeProbByLaneInfo1 ==
  LM_VSLFntPathBaseC1 : Inport
  Constant5 : Constant  Value=0.015  OutDataTypeStr=single
  Relational Operator5 : RelationalOperator  Operator=>  OutDataTypeStr=boolean  RndMeth=Nearest
  DIR_LaneChgRigByLineC1Valid : Outport
  wires:
  Relational Operator5/1 -> DIR_LaneChgRigByLineC1Valid/1  "DIR_LaneChgRigByLineC1Valid"
  LM_VSLFntPathBaseC1/1 -> Relational Operator5/1
  Constant5/1 -> Relational Operator5/2

== system PubIfDecisionLM_MDL/Subsystem2/DIR/DrivingIntentionRecognition1/DIR_LaneChangeProbCalc/DIR_LaneChangeRightProbCalc/If Action Subsystem1/DIR_LaneChgLeProbCalc ==
  DIR_LC2RigProbBySteer : Inport
  DIR_LC2RjgProbByLaneBorder : Inport  Port=2
  DIR_LaneChgRigByLineC1Valid : Inport  Port=3
  Logical Operator : Logic  Operator=OR  AllPortsSameDT=off  OutDataTypeStr=boolean
  Logical Operator1 : Logic  AllPortsSameDT=off  OutDataTypeStr=boolean
  DIR_tLC2RigValid : Outport
  wires:
  DIR_LaneChgRigByLineC1Valid/1 -> Logical Operator1/2
  Logical Operator/1 -> Logical Operator1/1
  DIR_LC2RjgProbByLaneBorder/1 -> Logical Operator/2
  DIR_LC2RigProbBySteer/1 -> Logical Operator/1
  Logical Operator1/1 -> DIR_tLC2RigValid/1  "DIR_tLC2RigValid"

== system PubIfDecisionLM_MDL/Subsystem2/DIR/DrivingIntentionRecognition1/DIR_LaneChangeProbCalc/DIR_LaneChangeRightProbCalc/If Action Subsystem1/DIR_LaneChgLeProbCalcBySteer ==
  SteerWheelAngle : Inport
  SteerWheelAngleSign : Inport  Port=2
  DIR_EgoVehOnLineValid : Inport  Port=3
  vxvRefMs : Inport  Port=4
  If : If  IfExpression=u1 ~= 0
  If Action Subsystem : Subsystem  TreatAsAtomicUnit=on
  If Action Subsystem1 : Subsystem  TreatAsAtomicUnit=on
  Merge : Merge
  DIR_LaneChgRigBySteerValid : Outport
  wires:
  Merge/1 -> DIR_LaneChgRigBySteerValid/1  "DIR_LaneChgRigBySteerValid"
  If Action Subsystem1/1(DIR_LaneChgRigBySteerValid) -> Merge/2
  If Action Subsystem/1(DIR_LaneChgRigBySteerValid) -> Merge/1
  vxvRefMs/1 -> If Action Subsystem/3(vxvRefMs), If Action Subsystem1/3(vxvRefMs)
  SteerWheelAngleSign/1 -> If Action Subsystem/2(SteerWheelAngleSign), If Action Subsystem1/2(SteerWheelAngleSign)
  SteerWheelAngle/1 -> If Action Subsystem/1(SteerWheelAngle), If Action Subsystem1/1(SteerWheelAngle)
  If/2 -> If Action Subsystem1/Action
  If/1 -> If Action Subsystem/Action
  DIR_EgoVehOnLineValid/1 -> If/1

== system PubIfDecisionLM_MDL/Subsystem2/LM_EML/LM_EMLFntPath1/LM_EMLKapAdjVal/LM_EMLMinKapWithin3Sec/If Action Subsystem1/LM_EMLKapBufMinValSearch ==
  LM_EMLKapBuf : Inport
  P_LM_EMLHistKapRcdBufSize : Inport  Port=2
  Abs : Abs
  Abs1 : Abs
  Compare To Constant : simulink/Logic and Bit Operations/Compare To Constant  relop===  const=1  OutDataTypeStr=boolean
  For Iterator : ForIterator  IterationSource=external  IterationLimit=30
  Index Vector : MultiPortSwitch  Inputs=1
  Relational Operator : RelationalOperator  Operator=<=  OutDataTypeStr=boolean  RndMeth=Simplest
  Switch : Switch  Criteria=u2 ~= 0
  Switch1 : Switch  Criteria=u2 ~= 0
  Unit Delay : UnitDelay  SampleTime=-1  HasFrameUpgradeWarning=on
  LM_EMLMinKap : Outport
  wires:
  LM_EMLKapBuf/1 -> Index Vector/2
  For Iterator/1 -> Compare To Constant/1, Index Vector/1
  Compare To Constant/1 -> Switch/2
  Index Vector/1 -> Switch1/1, Abs/1, Switch/1
  Switch/1 -> LM_EMLMinKap/1, Unit Delay/1  "LM_EMLMinKap"
  Abs/1 -> Relational Operator/1
  Abs1/1 -> Relational Operator/2
  Relational Operator/1 -> Switch1/2
  Unit Delay/1 -> Switch1/3, Abs1/1
  Switch1/1 -> Switch/3
  P_LM_EMLHistKapRcdBufSize/1 -> For Iterator/1

== system PubIfDecisionLM_MDL/Subsystem2/LM_Fusion1/LM_FusRatioCalc/LM_Fusion_EO/LM_FusEVORatioCalc/LM_Fusion_FntPathK/LM_FusEOFntPath1 ==
  vxvRefMs : Inport
  LM_EMLFntPath1Quality : Inport  Port=2
  LM_OTLFntPath1Qulity : Inport  Port=3
  LM_FusEOFusType : Inport  Port=4
  Constant : Constant  Value=0  OutDataTypeStr=single
  Constant1 : Constant  Value=0  OutDataTypeStr=single
  Constant2 : Constant  Value=0  OutDataTypeStr=single
  If : If  IfExpression=u1 == 2
  If Action Subsystem : Subsystem  TreatAsAtomicUnit=on
  If Action Subsystem1 : Subsystem  TreatAsAtomicUnit=on
  Merge : Merge
  Merge1 : Merge
  LM_FusEOFntPath1EMLK : Outport
  LM_FusEOFntPath1VSLK : Outport  Port=2
  LM_FusEOFntPath1OTLK : Outport  Port=3
  LM_FusEOFntPath1RELK : Outport  Port=4
  LM_FusEOFntPath1MALK : Outport  Port=5
  wires:
  Constant1/1 -> LM_FusEOFntPath1RELK/1  "LM_FusEOFntPath1RELK"
  Constant/1 -> LM_FusEOFntPath1VSLK/1  "LM_FusEOFntPath1VSLK"
  Constant2/1 -> LM_FusEOFntPath1MALK/1  "LM_FusEOFntPath1MALK"
  LM_FusEOFusType/1 -> If/1
  If/1 -> If Action Subsystem/Action
  If/2 -> If Action Subsystem1/Action
  vxvRefMs/1 -> If Action Subsystem1/1(vxvRefMs)
  LM_EMLFntPath1Quality/1 -> If Action Subsystem1/2(LM_EMLFntPath1Quality)
  LM_OTLFntPath1Qulity/1 -> If Action Subsystem1/3(LM_OTLFntPath1Qulity)
  If Action Subsystem/1(LM_FusEOFntPath1EMLK) -> Merge/1
  If Action Subsystem1/1(LM_FusEOFntPath1EMLK) -> Merge/2
  If Action Subsystem/2(LM_FusEOFntPath1OTLK) -> Merge1/1
  If Action Subsystem1/2(LM_FusEOFntPath1OTLK) -> Merge1/2
  Merge/1 -> LM_FusEOFntPath1EMLK/1
  Merge1/1 -> LM_FusEOFntPath1OTLK/1

== system PubIfDecisionLM_MDL/Subsystem2/LM_Fusion1/LM_FusRatioCalc/LM_Fusion_EO/LM_FusEVORatioCalc/LM_Fusion_FntPathK/LM_FusEOFntPath2 ==
  vxvRefMs : Inport
  LM_FusEOFusType : Inport  Port=2
  LM_EMLFntPath2Quality : Inport  Port=3
  LM_OTLFntPath2Qulity : Inport  Port=4
  Constant3 : Constant  Value=0  OutDataTypeStr=single
  Constant4 : Constant  Value=0  OutDataTypeStr=single
  Constant5 : Constant  Value=0  OutDataTypeStr=single
  If : If  IfExpression=u1 == 2
  If Action Subsystem : Subsystem  TreatAsAtomicUnit=on
  If Action Subsystem1 : Subsystem  TreatAsAtomicUnit=on
  Merge : Merge
  Merge1 : Merge
  LM_FusEOFntPath2EMLK : Outport
  LM_FusEOFntPath2VSLK : Outport  Port=2
  LM_FusEOFntPath2OTLK : Outport  Port=3
  LM_FusEOFntPath2RELK : Outport  Port=4
  LM_FusEOFntPath2MALK : Outport  Port=5
  wires:
  Constant5/1 -> LM_FusEOFntPath2MALK/1  "LM_FusEOFntPath2MALK"
  Constant3/1 -> LM_FusEOFntPath2VSLK/1  "LM_FusEOFntPath2VSLK"
  Constant4/1 -> LM_FusEOFntPath2RELK/1  "LM_FusEOFntPath2RELK"
  If/2 -> If Action Subsystem1/Action
  If/1 -> If Action Subsystem/Action
  LM_FusEOFusType/1 -> If/1
  vxvRefMs/1 -> If Action Subsystem1/1(vxvRefMs)
  LM_EMLFntPath2Quality/1 -> If Action Subsystem1/2(LM_EMLFntPath2Quality)
  LM_OTLFntPath2Qulity/1 -> If Action Subsystem1/3(LM_OTLFntPath2Qulity)
  If Action Subsystem/1(LM_FusEOFntPath2EMLK) -> Merge/1
  If Action Subsystem1/1(LM_FusEOFntPath2EMLK) -> Merge/2
  If Action Subsystem/2(LM_FusEOFntPath2OTLK) -> Merge1/1
  If Action Subsystem1/2(LM_FusEOFntPath2OTLK) -> Merge1/2
  Merge/1 -> LM_FusEOFntPath2EMLK/1
  Merge1/1 -> LM_FusEOFntPath2OTLK/1

== system PubIfDecisionLM_MDL/Subsystem2/LM_Fusion1/LM_FusRatioCalc/LM_Fusion_EO/LM_FusEVORatioCalc/LM_Fusion_FntPathK/LM_FusEOFntPath3 ==
  LM_FusEOFusType : Inport
  LM_EMLFntPath3Quality : Inport  Port=2
  LM_OTLFntPath3Qulity : Inport  Port=3
  Constant1 : Constant  Value=0  OutDataTypeStr=single
  Constant4 : Constant  Value=0  OutDataTypeStr=single
  Constant5 : Constant  Value=0  OutDataTypeStr=single
  If : If  IfExpression=u1 == 2
  If Action Subsystem : Subsystem  TreatAsAtomicUnit=on
  If Action Subsystem1 : Subsystem  TreatAsAtomicUnit=on
  Merge : Merge
  Merge1 : Merge
  LM_FusEOFntPath3EMLK : Outport
  LM_FusEOFntPath3VSLK : Outport  Port=2
  LM_FusEOFntPath3OTLK : Outport  Port=3
  LM_FusEOFntPath3RELK : Outport  Port=4
  LM_FusEOFntPath3MALK : Outport  Port=5
  wires:
  Constant1/1 -> LM_FusEOFntPath3VSLK/1  "LM_FusEOFntPath3VSLK"
  Constant5/1 -> LM_FusEOFntPath3MALK/1  "LM_FusEOFntPath3MALK"
  Constant4/1 -> LM_FusEOFntPath3RELK/1  "LM_FusEOFntPath3RELK"
  If/1 -> If Action Subsystem/Action
  If/2 -> If Action Subsystem1/Action
  If Action Subsystem/2(LM_FusEOFntPath3OTLK) -> Merge1/1
  LM_FusEOFusType/1 -> If/1
  If Action Subsystem1/2(LM_FusEOFntPath3OTLK) -> Merge1/2
  If Action Subsystem1/1(LM_FusEOFntPath3EMLK) -> Merge/2
  If Action Subsystem/1(LM_FusEOFntPath3EMLK) -> Merge/1
  Merge/1 -> LM_FusEOFntPath3EMLK/1
  Merge1/1 -> LM_FusEOFntPath3OTLK/1
  LM_EMLFntPath3Quality/1 -> If Action Subsystem1/1(LM_EMLFntPath3Quality)
  LM_OTLFntPath3Qulity/1 -> If Action Subsystem1/2(LM_OTLFntPath3Qulity)

== system PubIfDecisionLM_MDL/Subsystem2/LM_Fusion1/LM_FusRatioCalc/LM_Fusion_EO/LM_FusEVORatioCalc/LM_Fusion_FntPathK/LM_FusEOFusTypeCalc ==
  note: 完全用车道线场景：当车道线很好的时候可以完全用车道线，否则为了增加道路模型鲁棒性对三个道路模型加权平均
      | 1. 丢失车道数<=1
      | 2. 车道线质量大于0.65
      | 3. 第一段道路模型距离-VSL基础距离<=8m
  note: 0 Fus
      | 1 All VSL
      | 2 All EML
  DIR_TurnLeftValid : Inport
  DIR_TurnRightValid : Inport  Port=2
  DIR_LC2LeValid : Inport  Port=3
  DIR_LC2RigValid : Inport  Port=4
  Constant1 : Constant  Value=0  OutDataTypeStr=uint8
  Constant5 : Constant  Value=2  OutDataTypeStr=uint8
  Logical Operator1 : Logic  Operator=OR  Inputs=4  AllPortsSameDT=off  OutDataTypeStr=boolean
  Switch : Switch  Criteria=u2 ~= 0
  LM_FusEOFusType : Outport
  wires:
  Constant5/1 -> Switch/1
  Constant1/1 -> Switch/3
  Switch/1 -> LM_FusEOFusType/1  "LM_FusEOFusType"
  Logical Operator1/1 -> Switch/2  "LM_FusEVOAllEMLflg"
  DIR_TurnRightValid/1 -> Logical Operator1/2
  DIR_TurnLeftValid/1 -> Logical Operator1/1
  DIR_LC2LeValid/1 -> Logical Operator1/3
  DIR_LC2RigValid/1 -> Logical Operator1/4

== system PubIfDecisionLM_MDL/Subsystem2/LM_Fusion1/LM_FusRatioCalc/LM_Fusion_EV/LM_FusEMLAndVSLRatioCalc/LM_Fusion_FntPathK/LM_EVF_DeviationCalc ==
  LM_VSLFntPath1P : Inport
  LM_EMLFntPath1P : Inport  Port=2
  Abs : Abs
  Constant : Constant  Value=P_LM_FusEVDifC2Thre
  Constant2 : Constant  Value=P_LM_FusParC2Index  OutDataTypeStr=uint8
  Index Vector : MultiPortSwitch  Inputs=1
  Index Vector1 : MultiPortSwitch  Inputs=1
  Relational Operator : RelationalOperator  OutDataTypeStr=boolean  RndMeth=Nearest
  Subtract : Sum  Inputs=+-
  LM_FusEVdiffValid : Outport
  wires:
  Relational Operator/1 -> LM_FusEVdiffValid/1  "LM_FusEVdiffValid"
  Constant/1 -> Relational Operator/2
  Subtract/1 -> Abs/1
  LM_VSLFntPath1P/1 -> Index Vector1/2
  LM_EMLFntPath1P/1 -> Index Vector/2
  Index Vector/1 -> Subtract/1
  Index Vector1/1 -> Subtract/2
  Constant2/1 -> Index Vector1/1, Index Vector/1
  Abs/1 -> Relational Operator/1

== system PubIfDecisionLM_MDL/Subsystem2/LM_Fusion1/LM_FusRatioCalc/LM_Fusion_EVO/LM_FusEVORatioCalc/LM_Fusion_FntPathK/LM_FusEVOFntPath1 ==
  LM_EMLFntPath1Quality : Inport
  LM_VSLFntPath1Quality : Inport  Port=2
  LM_VSLBaseDis : Inport  Port=3
  LM_OTLFntPath1Qulity : Inport  Port=4
  LM_ComLineLostNum : Inport  Port=5
  LM_FntPath1Dis : Inport  Port=6
  vxvRefMs : Inport  Port=7
  DIR_TurnLeftValid : Inport  Port=8
  DIR_TurnRightValid : Inport  Port=9
  DIR_LC2LeValid : Inport  Port=10
  DIR_LC2RigValid : Inport  Port=11
  Constant : Constant  Value=0  OutDataTypeStr=single
  Constant1 : Constant  Value=0  OutDataTypeStr=single
  If : If  IfExpression=u1 == 1  ElseIfExpressions=u1 ==2
  If Action Subsystem1 : Subsystem  TreatAsAtomicUnit=on
  LM_FUS_EVOFEMLKAdju : Subsystem
  LM_FusEVOFntPath1AllEML : Subsystem  TreatAsAtomicUnit=on
  LM_FusEVOFntPath1AllVSL : Subsystem  TreatAsAtomicUnit=on
  LM_FusEVO_AllVSLJudge : Subsystem
  Merge : Merge  Inputs=3
  Merge1 : Merge  Inputs=3
  Merge2 : Merge  Inputs=3
  LM_FusEVOFntPath1EMLK : Outport
  LM_FusEVOFntPath1VSLK : Outport  Port=2
  LM_FusEVOFntPath1OTLK : Outport  Port=3
  LM_FusEVOFntPath1RELK : Outport  Port=4
  LM_FusEVOFntPath1MALK : Outport  Port=5
  wires:
  LM_FusEVO_AllVSLJudge/1(LM_FusEVOFusType) -> If/1
  If/1 -> LM_FusEVOFntPath1AllVSL/Action
  If/3 -> If Action Subsystem1/Action
  LM_VSLFntPath1Quality/1 -> If Action Subsystem1/1(LM_VSLFntPath1Quality), LM_FusEVO_AllVSLJudge/6(LM_VSLFntPath1Quality)
  LM_VSLBaseDis/1 -> LM_FusEVO_AllVSLJudge/1(LM_VSLBaseDis)
  LM_ComLineLostNum/1 -> LM_FusEVO_AllVSLJudge/2(LM_ComLineLostNum)
  LM_FntPath1Dis/1 -> LM_FusEVO_AllVSLJudge/3(LM_FntPath1Dis)
  vxvRefMs/1 -> [vxvRefMs], If Action Subsystem1/2(vxvRefMs)
  LM_EMLFntPath1Quality/1 -> [LM_EMLFntPath1Quality], If Action Subsystem1/3(LM_EMLFntPath1Quality)
  LM_OTLFntPath1Qulity/1 -> If Action Subsystem1/4(LM_OTLFntPath1Qulity)
  LM_FusEVOFntPath1AllVSL/1(LM_FusEVOFntPath1EMLK) -> Merge/1
  If Action Subsystem1/1(LM_FusEVOFntPath1EMLK) -> Merge/3
  LM_FUS_EVOFEMLKAdju/1(LM_FusEVOFntPath1EMLK) -> LM_FusEVOFntPath1EMLK/1  "LM_FusEVOFntPath1EMLK"
  LM_FusEVOFntPath1AllVSL/2(LM_FusEVOFntPath1VSLK) -> Merge1/1
  If Action Subsystem1/2(LM_FusEVOFntPath1VSLK) -> Merge1/3
  LM_FUS_EVOFEMLKAdju/2(LM_FusEVOFntPath1VSLK) -> LM_FusEVOFntPath1VSLK/1  "LM_FusEVOFntPath1VSLK"
  LM_FusEVOFntPath1AllVSL/3(LM_FusEVOFntPath1OTLK) -> Merge2/1
  If Action Subsystem1/3(LM_FusEVOFntPath1OTLK) -> Merge2/3
  LM_FUS_EVOFEMLKAdju/3(LM_FusEVOFntPath1OTLK) -> LM_FusEVOFntPath1OTLK/1  "LM_FusEVOFntPath1OTLK"
  Constant/1 -> LM_FusEVOFntPath1RELK/1  "LM_FusEVOFntPath1RELK"
  Constant1/1 -> LM_FusEVOFntPath1MALK/1  "LM_FusEVOFntPath1MALK"
  DIR_TurnLeftValid/1 -> LM_FusEVO_AllVSLJudge/4(DIR_TurnLeftValid)
  DIR_TurnRightValid/1 -> LM_FusEVO_AllVSLJudge/5(DIR_TurnRightValid)
  If/2 -> LM_FusEVOFntPath1AllEML/Action
  DIR_LC2LeValid/1 -> [DIR_LC2LeValid], If Action Subsystem1/5(DIR_LC2LeValid)
  DIR_LC2RigValid/1 -> [DIR_LC2RigValid], If Action Subsystem1/6(DIR_LC2RigValid)
  LM_FusEVOFntPath1AllEML/1(LM_FusEVOFntPath1EMLK) -> Merge/2
  LM_FusEVOFntPath1AllEML/2(LM_FusEVOFntPath1VSLK) -> Merge1/2
  LM_FusEVOFntPath1AllEML/3(LM_FusEVOFntPath1OTLK) -> Merge2/2
  Merge/1 -> LM_FUS_EVOFEMLKAdju/5(LM_FusEVOFntPath1EMLKBefAdju)
  Merge1/1 -> LM_FUS_EVOFEMLKAdju/6(LM_FusEVOFntPath1VSLKBefAdju)
  Merge2/1 -> LM_FUS_EVOFEMLKAdju/7(LM_FusEVOFntPath1OTLKBefAdju)
  [vxvRefMs] -> LM_FUS_EVOFEMLKAdju/4(vxvRefMs)
  [DIR_LC2RigValid] -> LM_FUS_EVOFEMLKAdju/3(DIR_LC2RigValid)
  [DIR_LC2LeValid] -> LM_FUS_EVOFEMLKAdju/2(DIR_LC2LeValid)
  [LM_EMLFntPath1Quality] -> LM_FUS_EVOFEMLKAdju/1(LM_EMLFntPath1Quality)

== system PubIfDecisionLM_MDL/Subsystem2/LM_Fusion1/LM_FusRatioCalc/LM_Fusion_EVO/LM_FusEVORatioCalc/LM_Fusion_FntPathK/LM_FusEVOFntPath2 ==
  LM_ComLineLostNum : Inport
  LM_EMLFntPath2Quality : Inport  Port=2
  LM_VSLFntPath2Quality : Inport  Port=3
  LM_OTLFntPath2Qulity : Inport  Port=4
  DIR_TurnLeftValid : Inport  Port=5
  DIR_TurnRightValid : Inport  Port=6
  LM_VSLBaseDis : Inport  Port=7
  LM_FntPath2Dis : Inport  Port=8
  vxvRefMs : Inport  Port=9
  DIR_LC2LeValid : Inport  Port=10
  DIR_LC2RigValid : Inport  Port=11
  Constant3 : Constant  Value=0  OutDataTypeStr=single
  Constant4 : Constant  Value=0  OutDataTypeStr=single
  If : If  IfExpression=u1 == 1  ElseIfExpressions=u1 == 2
  If Action Subsystem : Subsystem  TreatAsAtomicUnit=on
  If Action Subsystem1 : Subsystem  TreatAsAtomicUnit=on
  If Action Subsystem2 : Subsystem  TreatAsAtomicUnit=on
  LM_FusEVO_AllVSLJudge : Subsystem
  Merge : Merge  Inputs=3
  Merge1 : Merge  Inputs=3
  Merge2 : Merge  Inputs=3
  LM_FusEVOFntPath2EMLK : Outport
  LM_FusEVOFntPath2VSLK : Outport  Port=2
  LM_FusEVOFntPath2OTLK : Outport  Port=3
  LM_FusEVOFntPath2RELK : Outport  Port=4
  LM_FusEVOFntPath2MALK : Outport  Port=5
  wires:
  Constant3/1 -> LM_FusEVOFntPath2RELK/1  "LM_FusEVOFntPath2RELK"
  Constant4/1 -> LM_FusEVOFntPath2MALK/1  "LM_FusEVOFntPath2MALK"
  LM_FusEVO_AllVSLJudge/1(LM_FusEVOFntPath2FusType) -> If/1
  If Action Subsystem1/3(LM_FusEVOFntPath2OTLK) -> Merge2/3
  If Action Subsystem/3(LM_FusEVOFntPath2OTLK) -> Merge2/1
  If Action Subsystem1/2(LM_FusEVOFntPath2VSLK) -> Merge1/3
  If Action Subsystem/2(LM_FusEVOFntPath2VSLK) -> Merge1/1
  If Action Subsystem1/1(LM_FusEVOFntPath2EMLK) -> Merge/3
  If Action Subsystem/1(LM_FusEVOFntPath2EMLK) -> Merge/1
  If/1 -> If Action Subsystem/Action
  If/3 -> If Action Subsystem1/Action
  Merge/1 -> LM_FusEVOFntPath2EMLK/1  "LM_FusEVOFntPath1EMLK"
  Merge1/1 -> LM_FusEVOFntPath2VSLK/1  "LM_FusEVOFntPath1VSLK"
  Merge2/1 -> LM_FusEVOFntPath2OTLK/1  "LM_FusEVOFntPath1OTLK"
  LM_OTLFntPath2Qulity/1 -> If Action Subsystem1/3(LM_OTLFntPath2Qulity)
  LM_VSLFntPath2Quality/1 -> If Action Subsystem1/2(LM_VSLFntPath2Quality)
  LM_EMLFntPath2Quality/1 -> LM_FusEVO_AllVSLJudge/6(LM_VSLFntPath2Quality), If Action Subsystem1/1(LM_EMLFntPath2Quality)
  LM_ComLineLostNum/1 -> LM_FusEVO_AllVSLJudge/1(LM_ComLineLostNum)
  If/2 -> If Action Subsystem2/Action
  DIR_TurnLeftValid/1 -> LM_FusEVO_AllVSLJudge/2(DIR_TurnLeftValid)
  DIR_TurnRightValid/1 -> LM_FusEVO_AllVSLJudge/3(DIR_TurnRightValid)
  LM_FntPath2Dis/1 -> LM_FusEVO_AllVSLJudge/5(LM_FntPath2Dis)
  LM_VSLBaseDis/1 -> LM_FusEVO_AllVSLJudge/4(LM_VSLBaseDis)
  vxvRefMs/1 -> If Action Subsystem1/4(vxvRefMs)
  DIR_LC2LeValid/1 -> If Action Subsystem1/5(DIR_LC2LeValid)
  DIR_LC2RigValid/1 -> If Action Subsystem1/6(DIR_LC2RigValid)
  If Action Subsystem2/1(LM_FusEVOFntPath2EMLK) -> Merge/2
  If Action Subsystem2/2(LM_FusEVOFntPath2VSLK) -> Merge1/2
  If Action Subsystem2/3(LM_FusEVOFntPath2OTLK) -> Merge2/2

== system PubIfDecisionLM_MDL/Subsystem2/LM_Fusion1/LM_FusRatioCalc/LM_Fusion_EVO/LM_FusEVORatioCalc/LM_Fusion_FntPathK/LM_FusEVOFntPath3 ==
  LM_ComLineLostNum : Inport
  LM_EMLFntPath3Quality : Inport  Port=2
  LM_VSLFntPath3Quality : Inport  Port=3
  LM_OTLFntPath3Quality : Inport  Port=4
  DIR_TurnLeftValid : Inport  Port=5
  DIR_TurnRightValid : Inport  Port=6
  vxvRefMs : Inport  Port=7
  DIR_LC2LeValid : Inport  Port=8
  DIR_LC2RigValid : Inport  Port=9
  Constant : Constant  Value=0  OutDataTypeStr=single
  Constant1 : Constant  Value=0  OutDataTypeStr=single
  If : If  IfExpression=u1 == 1  ElseIfExpressions=u1 == 2
  If Action Subsystem : Subsystem  TreatAsAtomicUnit=on
  If Action Subsystem1 : Subsystem  TreatAsAtomicUnit=on
  If Action Subsystem2 : Subsystem  TreatAsAtomicUnit=on
  LM_FusEVO_AllVSLJudge : Subsystem
  Merge : Merge  Inputs=3
  Merge1 : Merge  Inputs=3
  Merge2 : Merge  Inputs=3
  LM_FusEVOFntPath3EMLK : Outport
  LM_FusEVOFntPath3VSLK : Outport  Port=2
  LM_FusEVOFntPath3OTLK : Outport  Port=3
  LM_FusEVOFntPath3RELK : Outport  Port=4
  LM_FusEVOFntPath3MALK : Outport  Port=5
  wires:
  Constant/1 -> LM_FusEVOFntPath3RELK/1  "LM_FusEVOFntPath3RELK"
  Constant1/1 -> LM_FusEVOFntPath3MALK/1  "LM_FusEVOFntPath3MALK"
  If/1 -> If Action Subsystem/Action
  LM_FusEVO_AllVSLJudge/1(LM_FusEVOFntPath3FusType) -> If/1
  LM_ComLineLostNum/1 -> LM_FusEVO_AllVSLJudge/1(LM_ComLineLostNum)
  LM_OTLFntPath3Quality/1 -> If Action Subsystem1/3(LM_OTLFntPath3Qulity)
  If/3 -> If Action Subsystem1/Action
  If Action Subsystem1/3(LM_FusEVOFntPath3OTLK) -> Merge2/3
  LM_EMLFntPath3Quality/1 -> If Action Subsystem1/1(LM_EMLFntPath3Quality)
  If Action Subsystem1/1(LM_FusEVOFntPath3EMLK) -> Merge/3
  If Action Subsystem1/2(LM_FusEVOFntPath3VSLK) -> Merge1/3
  If Action Subsystem/1(LM_FusEVOFntPath3EMLK) -> Merge/1
  If Action Subsystem/2(LM_FusEVOFntPath3VSLK) -> Merge1/1
  If Action Subsystem/3(LM_FusEVOFntPath3OTLK) -> Merge2/1
  Merge/1 -> LM_FusEVOFntPath3EMLK/1  "LM_FusEVOFntPath3EMLK"
  Merge1/1 -> LM_FusEVOFntPath3VSLK/1  "LM_FusEVOFntPath3VSLK"
  Merge2/1 -> LM_FusEVOFntPath3OTLK/1  "LM_FusEVOFntPath3OTLK"
  If/2 -> If Action Subsystem2/Action
  DIR_TurnRightValid/1 -> LM_FusEVO_AllVSLJudge/3(DIR_TurnRightValid)
  DIR_TurnLeftValid/1 -> LM_FusEVO_AllVSLJudge/2(DIR_TurnLeftValid)
  vxvRefMs/1 -> If Action Subsystem1/4(vxvRefMs)
  DIR_LC2LeValid/1 -> If Action Subsystem1/5(DIR_LC2LeValid)
  DIR_LC2RigValid/1 -> If Action Subsystem1/6(DIR_LC2RigValid)
  If Action Subsystem2/1(LM_FusEVOFntPath3EMLK) -> Merge/2
  If Action Subsystem2/2(LM_FusEVOFntPath3VSLK) -> Merge1/2
  If Action Subsystem2/3(LM_FusEVOFntPath3OTLK) -> Merge2/2
  LM_VSLFntPath3Quality/1 -> LM_FusEVO_AllVSLJudge/4(LM_VSLFntPath3Quality), If Action Subsystem1/2(LM_VSLFntPath3Quality)
